simulink model "arduino_lab_R2014a"  (R2014a)
settings: Solver=ode45  StartTime=0.0  StopTime=500  RelTol=1e-3
StartFcn:
  | clear all
libraries: realtime_pacer_lib x1
settings Model: CovSFcnEnable=on  Creator=johnh  LastModifiedBy=johnh
settings DataIOCC: LimitDataPoints=off  SaveFormat=StructureWithTime
settings DebuggingCC: MergeDetectMultiDrivingBlocksExec=error  SolverPrmCheckMsg=none  FrameProcessingCompatibilityMsg=error
settings HardwareCC: ProdBitPerPointer=64  ProdLargestAtomicFloat=Float  ProdIntDivRoundTo=Zero  ProdEndianess=LittleEndian  ProdHWDeviceType=Specified
settings ModelReferenceCC: PropagateSignalLabelsOutOfModel=on

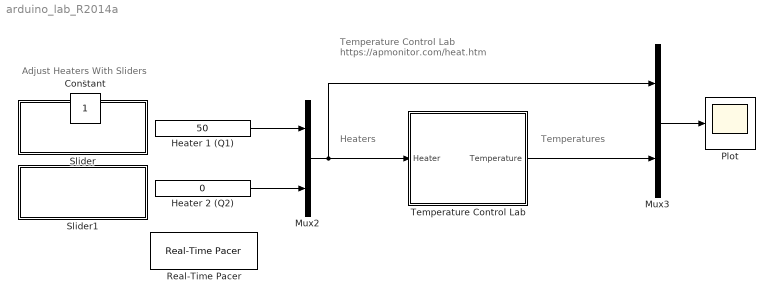
== system arduino_lab_R2014a ==
  note: Adjust Heaters With Sliders
  note: Temperature Control Lab
      | https://apmonitor.com/heat.htm
  note: Heaters
  note: Temperatures
  Heater 1 (Q1) : Constant  Value=50
  Heater 2 (Q2) : Constant  Value=0
  Mux2 : Mux  Inputs=2
  Mux3 : Mux  Inputs=2
  Plot : Scope
      settings: TimeRange=auto  LimitDataPoints=on  MaxDataPoints=5000  SaveToWorkspace=off  SaveName=ScopeData  YMin=-12.5  YMax=112.5  SampleTime=-1  DataFormat=Array
  Real-Time Pacer : realtime_pacer_lib/Real-Time Pacer  simTimePerRealTime=1
  Slider : Subsystem  Description=Replaced Block  mask(Replaced Block){}
      mask help: This block has been replaced with an empty subsystem because it used functionality that is unavailable in Simulink R2014a.
      mask Display: fprintf('Replaced: %s\n','Dashboard Widget')
  Slider1 : Subsystem  Description=Replaced Block  mask(Replaced Block){}
      mask help: This block has been replaced with an empty subsystem because it used functionality that is unavailable in Simulink R2014a.
      mask Display: fprintf('Replaced: %s\n','Dashboard Widget')
  Temperature Control Lab : Subsystem
      mask Display: image('tclab.png');
  1 : Constant  IOType=siggen
  Constant : Constant  IOType=siggen
  wires:
  Heater 1 (Q1)/1 -> Mux2/1
  Heater 2 (Q2)/1 -> Mux2/2
  Temperature Control Lab/1(Temperature) -> Mux3/2
  Mux3/1 -> Plot/1
  Mux2/1 -> Mux3/1, Temperature Control Lab/1(Heater)

== system arduino_lab_R2014a/Slider ==

== system arduino_lab_R2014a/Slider1 ==

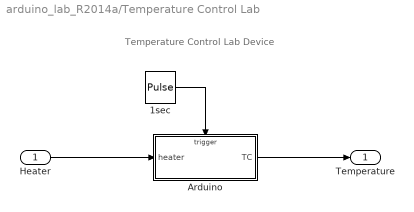
== system arduino_lab_R2014a/Temperature Control Lab ==
  note: Temperature Control Lab Device
  Heater : Inport
  1sec : DiscretePulseGenerator  PulseType=Time based  Period=1  PulseWidth=50
  Arduino : Subsystem  TreatAsAtomicUnit=on
  Temperature : Outport
  wires:
  1sec/1 -> Arduino/Trigger
  Arduino/1(TC) -> Temperature/1
  Heater/1 -> Arduino/1(heater)

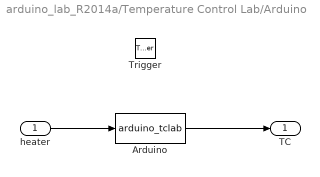
== system arduino_lab_R2014a/Temperature Control Lab/Arduino ==
  heater : Inport  LatchByDelayingOutsideSignal=on
  Trigger : TriggerPort
  Arduino : MATLABFcn  MATLABFcn=arduino_tclab
  TC : Outport  InitialOutput=[23 23]
  wires:
  heater/1 -> Arduino/1
  Arduino/1 -> TC/1
